simulink model "PlexonReceive"  (R2016a)
settings: Solver=FixedStepAuto  StartTime=0.0  StopTime=10.0  RelTol=1e-3
undefined symbols (not defined in the file or in its folder): sCoreParams
settings Model: Creator=rzelmann  LastModifiedBy=rzelmann
settings SolverCC: EnableConcurrentExecution=on  AutoInsertRateTranBlk=on
settings DataIOCC: SaveFormat=StructureWithTime
settings OptimizationCC: BlockReduction=off  OptimizeBlockIOStorage=off  BufferReuse=off  GlobalBufferReuse=off  ExpressionFolding=off  LocalBlockOutputs=off
settings HardwareCC: ProdBitPerPointer=32  ProdLargestAtomicFloat=None  ProdWordSize=32  ProdLongLongMode=on  ProdHWDeviceType=Generic->32-bit x86 compatible
settings RTWCC: SystemTargetFile=slrt.tlc  TemplateMakefile=slrt_default_tmf  Description=Simulink Real-Time  RTWCompilerOptimization=on

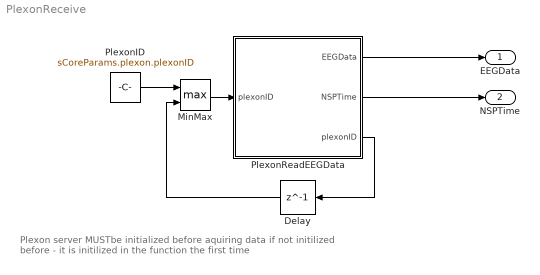
== system PlexonReceive ==
  note: Plexon server MUSTbe initialized before aquiring data
      | if not initilized before - it is  initilized in the function the first time
  Delay : Delay  DelayLength=1
  MinMax : MinMax  Function=max  Inputs=2
  PlexonID : Constant  Value=sCoreParams.plexon.plexonID
  PlexonReadEEGData : MATLAB Function  TreatAsAtomicUnit=on
  EEGData : Outport
  NSPTime : Outport  Port=2
  wires:
  PlexonReadEEGData/2(NSPTime) -> NSPTime/1
  PlexonReadEEGData/1(EEGData) -> EEGData/1
  PlexonID/1 -> MinMax/1
  MinMax/1 -> PlexonReadEEGData/1("plexonID ")
  PlexonReadEEGData/3(plexonID) -> Delay/1
  Delay/1 -> MinMax/2

== matlab function PlexonReceive/PlexonReadEEGData ==
  data: plexonID input; EEGData output; NSPTime output; plexonID output
function [EEGData, NSPTime, plexonID] = PlexonReadEEGData(plexonID)
%#codegen

[EEGData, NSPTime, plexonID]  = PlexonReadEEGData_EML(plexonID);
